simulink model "team_project_state_and_cds"  (R2023b)
settings: Solver=FixedStepAuto  StartTime=0.0  StopTime=inf  FixedStep=0.01  RelTol=1e-3  EnableMultiTasking=on
libraries: arduinolib x7
settings Model: ExtModeTrigDuration=2  Creator=권주성  LastModifiedBy=tkdle
settings OptimizationCC: EnhancedBackFolding=on  PassReuseOutputArgsAs=Individual arguments  ZeroExternalMemoryAtStartup=off  ZeroInternalMemoryAtStartup=off  MaxStackSize=64  OptimizeBlockOrder=speed  DifferentSizesBufferReuse=on  OptimizationCustomize=off  EfficientTunableParamExpr=on
settings DebuggingCC: ParameterTunabilityLossMsg=error
settings HardwareCC: ProdBitPerInt=16  ProdBitPerPointer=16  ProdBitPerSizeT=16  ProdBitPerPtrDiffT=16  ProdLargestAtomicFloat=None  ProdWordSize=8  ProdHWDeviceType=Atmel->AVR
settings SFSimCC: MATLABDynamicMemAlloc=off
settings RTWCC: Description=Embedded Coder  SystemTargetFile=ert.tlc  HardwareBoard=Arduino Mega ADK  TemplateMakefile=ert_default_tmf  Toolchain=Arduino AVR  BuildConfiguration=Faster Runs
settings CodeAppCC: ForceParamTrailComments=on  IgnoreCustomStorageClasses=off  OperatorAnnotations=on  SimulinkDataObjDesc=on  SFDataObjDesc=on  InsertBlockDesc=on
settings ERTTargetCC: SupportContinuousTime=on  SupportVariableSizeSignals=on  ExtModeTransport=3  ExtModeStaticAlloc=on  ExtModeAutomaticAllocSize=off  ExtModeStaticAllocSize=2048  ExtModeMexFile=ext_xcp  ExtModeIntrfLevel=Level2 - Open

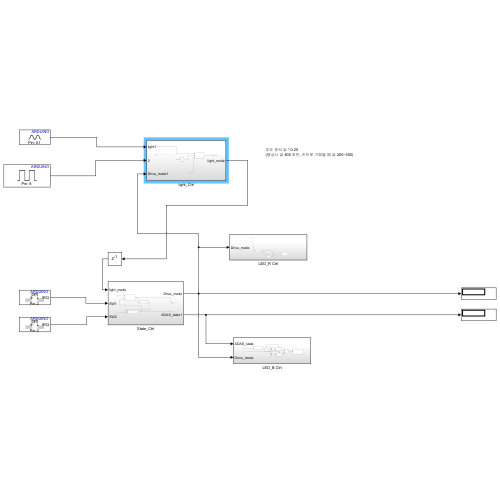
[thumbnail: Simulink's stored preview of the top-level diagram]
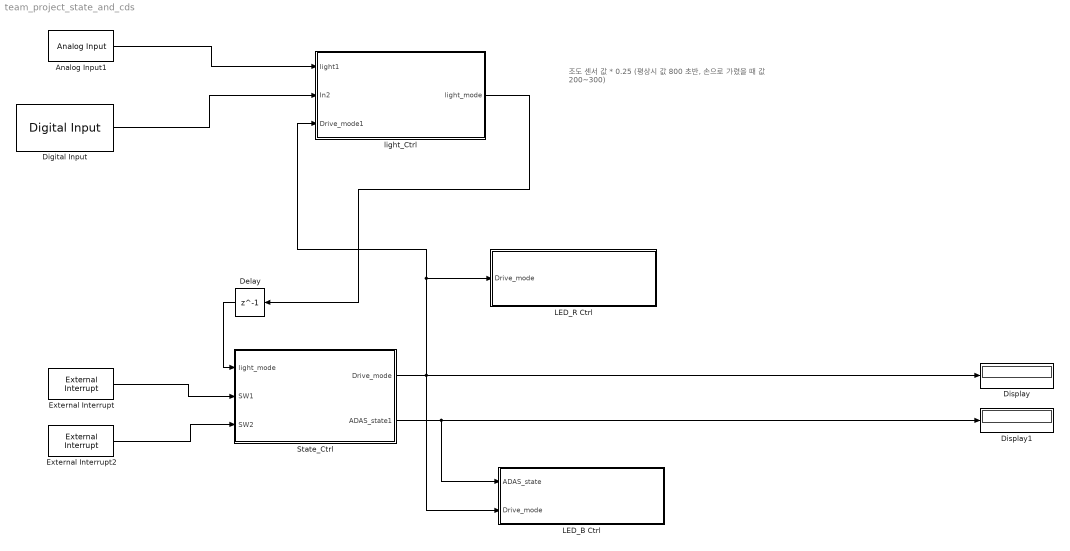
== system team_project_state_and_cds ==
  note: 조도 센서 값 * 0.25
      | (평상시 값 800 초반, 손으로 가렸을 때 값 200~300)
  Analog Input1 : arduinolib/Analog Input  pinNumber=1  ReadResultsOnly=off  ConversionTriggerSource=Software  ExternalTriggerType=uint32( 0 )  OutputDataType=uint16  EnableConversionCompleteNotify=off  EnableOuputStatus=off  SampleTime=-1  blockPlatform=arduino
  Delay : Delay  DelayLength=1
  Digital Input : arduinolib/Digital Input  pinNumber=8  mode=Default  Direction=input  SampleTime=0.1  blockPlatform=arduino
  Display : Display
  Display1 : Display
  External Interrupt : arduinolib/External Interrupt  Pin=2  PullUp=off  Mode=RISING  InterruptSimulationInput=off
  External Interrupt2 : arduinolib/External Interrupt  Pin=3  PullUp=off  Mode=RISING  InterruptSimulationInput=off
  LED_B Ctrl : Subsystem
  LED_R Ctrl : Subsystem
  State_Ctrl : Subsystem
  light_Ctrl : Subsystem
  wires:
  light_Ctrl/1(light_mode) -> Delay/1
  Digital Input/1 -> light_Ctrl/2(In2)
  Analog Input1/1 -> light_Ctrl/1(light1)
  Delay/1 -> State_Ctrl/1(light_mode)
  State_Ctrl/2(ADAS_state1) -> LED_B Ctrl/1(ADAS_state), Display1/1
  External Interrupt/1 -> State_Ctrl/2(SW1)
  External Interrupt2/1 -> State_Ctrl/3(SW2)
  State_Ctrl/1(Drive_mode) -> Display/1, light_Ctrl/3(Drive_mode1), LED_R Ctrl/1(Drive_mode), LED_B Ctrl/2(Drive_mode)

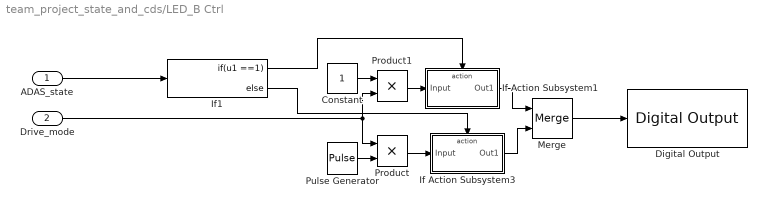
== system team_project_state_and_cds/LED_B Ctrl ==
  ADAS_state : Inport
  Drive_mode : Inport  Port=2
  Constant : Constant
  Digital Output : arduinolib/Digital Output  pinNumber=43  Direction=output  blockPlatform=arduino
  If Action Subsystem1 : Subsystem  TreatAsAtomicUnit=on
  If Action Subsystem3 : Subsystem  TreatAsAtomicUnit=on
  If1 : If  IfExpression=u1 ==1
  Merge : Merge
  Product : Product
  Product1 : Product
  Pulse Generator : DiscretePulseGenerator  PulseType=Time based  PulseWidth=50
  wires:
  If1/2 -> If Action Subsystem3/Action
  If Action Subsystem1/1(Out1) -> Merge/1
  ADAS_state/1 -> If1/1
  If1/1 -> If Action Subsystem1/Action
  Merge/1 -> Digital Output/1
  If Action Subsystem3/1(Out1) -> Merge/2
  Drive_mode/1 -> Product/1, Product1/2
  Pulse Generator/1 -> Product/2
  Constant/1 -> Product1/1
  Product1/1 -> If Action Subsystem1/1(Input)
  Product/1 -> If Action Subsystem3/1(Input)

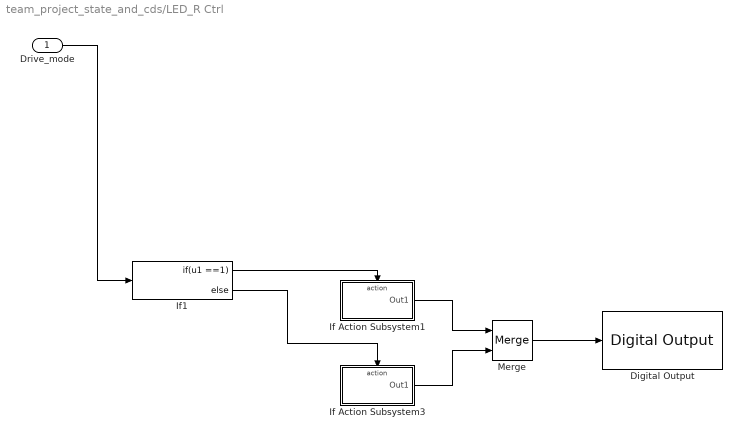
== system team_project_state_and_cds/LED_R Ctrl ==
  Drive_mode : Inport
  Digital Output : arduinolib/Digital Output  pinNumber=42  Direction=output  blockPlatform=arduino
  If Action Subsystem1 : Subsystem  TreatAsAtomicUnit=on
  If Action Subsystem3 : Subsystem  TreatAsAtomicUnit=on
  If1 : If  IfExpression=u1 ==1
  Merge : Merge
  wires:
  If1/2 -> If Action Subsystem3/Action
  If Action Subsystem1/1(Out1) -> Merge/1
  Drive_mode/1 -> If1/1
  If1/1 -> If Action Subsystem1/Action
  Merge/1 -> Digital Output/1
  If Action Subsystem3/1(Out1) -> Merge/2

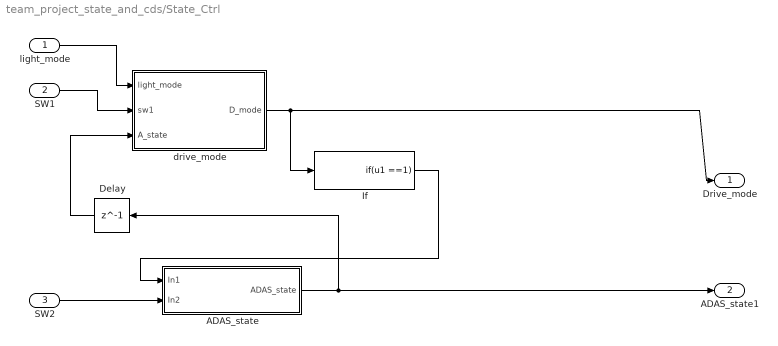
== system team_project_state_and_cds/State_Ctrl ==
  light_mode : Inport
  SW1 : Inport  Port=2
  SW2 : Inport  Port=3
  ADAS_state : Subsystem
  Delay : Delay  DelayLength=1
  If : If  IfExpression=u1 ==1  ShowElse=off
  drive_mode : Subsystem
  Drive_mode : Outport
  ADAS_state1 : Outport  Port=2
  wires:
  If/1 -> ADAS_state/1(In1)
  drive_mode/1(D_mode) -> If/1, Drive_mode/1
  SW2/1 -> ADAS_state/2(In2)
  ADAS_state/1(ADAS_state) -> Delay/1, ADAS_state1/1
  SW1/1 -> drive_mode/2(sw1)
  Delay/1 -> drive_mode/3(A_state)
  light_mode/1 -> drive_mode/1(light_mode)

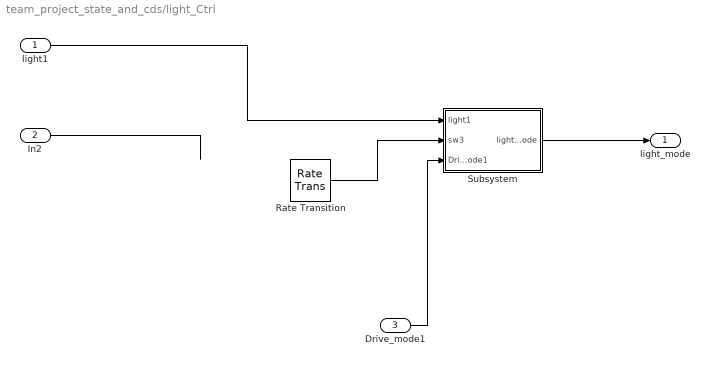
== system team_project_state_and_cds/light_Ctrl ==
  light1 : Inport
  In2 : Inport  Port=2
  Drive_mode1 : Inport  Port=3
  Rate Transition : RateTransition  Integrity=off  OutPortSampleTime=0.5
  Subsystem : Subsystem
  light_mode : Outport
  wires:
  ? -> Rate Transition/1
  In2/1 -> ?
  Rate Transition/1 -> Subsystem/2(sw3)
  Drive_mode1/1 -> Subsystem/3(Drive_mode1)
  light1/1 -> Subsystem/1(light1)
  Subsystem/1(light_mode) -> light_mode/1

== system team_project_state_and_cds/LED_B Ctrl/If Action Subsystem1 ==
  Input : Inport
  Action Port : ActionPort
  Out1 : Outport
  wires:
  Input/1 -> Out1/1

== system team_project_state_and_cds/LED_B Ctrl/If Action Subsystem3 ==
  Input : Inport
  Action Port : ActionPort
  Out1 : Outport
  wires:
  Input/1 -> Out1/1

== system team_project_state_and_cds/LED_R Ctrl/If Action Subsystem1 ==
  Action Port : ActionPort
  Constant : Constant
  Out1 : Outport
  wires:
  Constant/1 -> Out1/1

== system team_project_state_and_cds/LED_R Ctrl/If Action Subsystem3 ==
  Action Port : ActionPort
  Constant : Constant  Value=0
  Out1 : Outport
  wires:
  Constant/1 -> Out1/1

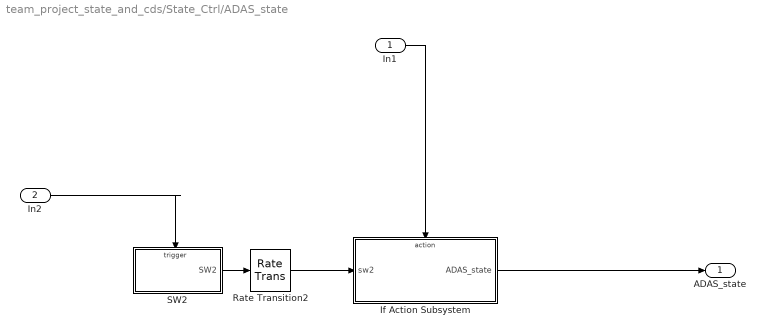
== system team_project_state_and_cds/State_Ctrl/ADAS_state ==
  In1 : Inport
  In2 : Inport  Port=2
  If Action Subsystem : Subsystem  TreatAsAtomicUnit=on
  Rate Transition2 : RateTransition  Integrity=off
  SW2 : Subsystem
  ADAS_state : Outport
  wires:
  Rate Transition2/1 -> If Action Subsystem/1(sw2)
  SW2/1(SW2) -> Rate Transition2/1
  In1/1 -> If Action Subsystem/Action
  In2/1 -> SW2/Trigger
  If Action Subsystem/1(ADAS_state) -> ADAS_state/1

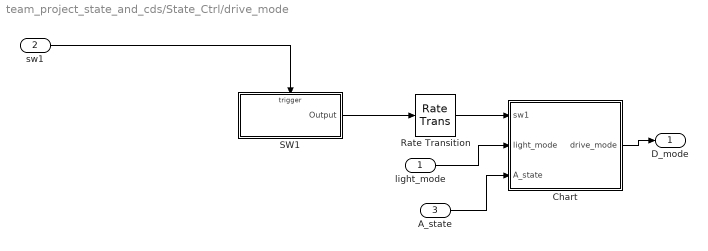
== system team_project_state_and_cds/State_Ctrl/drive_mode ==
  light_mode : Inport
  sw1 : Inport  Port=2
  A_state : Inport  Port=3
  Chart : Stateflow chart  TreatAsAtomicUnit=on
  Rate Transition : RateTransition  Integrity=off
  SW1 : Subsystem
  D_mode : Outport
  wires:
  SW1/1(Output) -> Rate Transition/1
  Rate Transition/1 -> Chart/1(sw1)
  Chart/1(drive_mode) -> D_mode/1
  sw1/1 -> SW1/Trigger
  A_state/1 -> Chart/3(A_state)
  light_mode/1 -> Chart/2(light_mode)

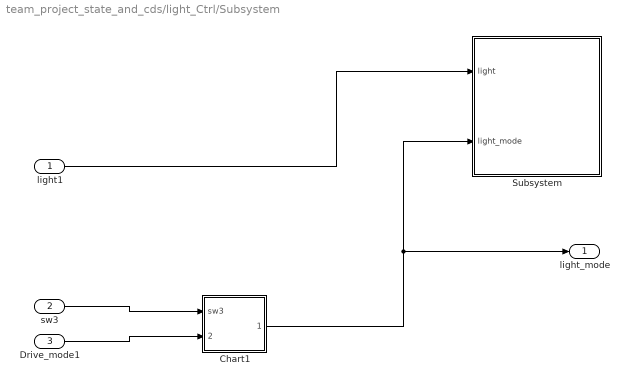
== system team_project_state_and_cds/light_Ctrl/Subsystem ==
  light1 : Inport
  sw3 : Inport  Port=2
  Drive_mode1 : Inport  Port=3
  Chart1 : Stateflow chart  TreatAsAtomicUnit=on
  Subsystem : Subsystem
  light_mode : Outport
  wires:
  Chart1/1(light_mode) -> Subsystem/2(light_mode), light_mode/1
  light1/1 -> Subsystem/1(light)
  sw3/1 -> Chart1/1(sw3)
  Drive_mode1/1 -> Chart1/2(Drive_mode)

== system team_project_state_and_cds/State_Ctrl/ADAS_state/If Action Subsystem ==
  sw2 : Inport
  Action Port : ActionPort
  Chart : Stateflow chart  TreatAsAtomicUnit=on
  ADAS_state : Outport
  wires:
  sw2/1 -> Chart/1(sw2)
  Chart/1(ADAS_state) -> ADAS_state/1

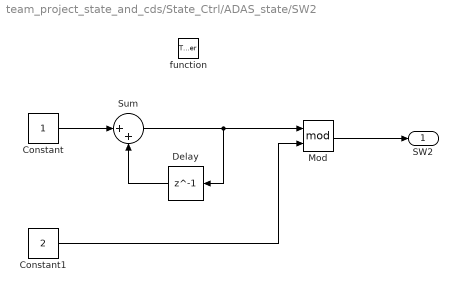
== system team_project_state_and_cds/State_Ctrl/ADAS_state/SW2 ==
  function : TriggerPort  TriggerType=function-call  VariantControl=(inherit)
  Constant : Constant
  Constant1 : Constant  Value=2
  Delay : Delay  DelayLength=1  InitialCondition=0
  Mod : Math  Operator=mod
  Sum : Sum  Inputs=|++
  SW2 : Outport
  wires:
  Sum/1 -> Delay/1, Mod/1
  Constant1/1 -> Mod/2
  Mod/1 -> SW2/1
  Constant/1 -> Sum/1
  Delay/1 -> Sum/2

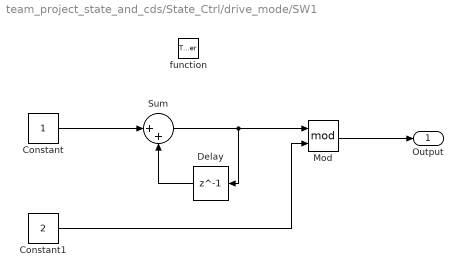
== system team_project_state_and_cds/State_Ctrl/drive_mode/SW1 ==
  function : TriggerPort  TriggerType=function-call  VariantControl=(inherit)
  Constant : Constant
  Constant1 : Constant  Value=2
  Delay : Delay  DelayLength=1
  Mod : Math  Operator=mod
  Sum : Sum  Inputs=|++
  Output : Outport
  wires:
  Constant/1 -> Sum/1
  Sum/1 -> Delay/1, Mod/1
  Constant1/1 -> Mod/2
  Delay/1 -> Sum/2
  Mod/1 -> Output/1

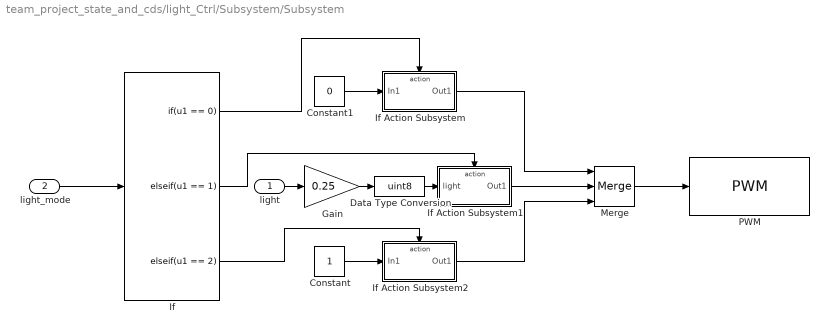
== system team_project_state_and_cds/light_Ctrl/Subsystem/Subsystem ==
  light : Inport
  light_mode : Inport  Port=2
  Constant : Constant
  Constant1 : Constant  Value=0
  Data Type Conversion : DataTypeConversion  OutDataTypeStr=uint8  SaturateOnIntegerOverflow=off  RndMeth=Floor
  Gain : Gain  Gain=0.25
  If : If  IfExpression=u1 == 0  ElseIfExpressions=u1 == 1, u1 == 2  ShowElse=off
  If Action Subsystem : Subsystem  TreatAsAtomicUnit=on
  If Action Subsystem1 : Subsystem  TreatAsAtomicUnit=on
  If Action Subsystem2 : Subsystem  TreatAsAtomicUnit=on
  Merge : Merge  Inputs=3
  PWM : arduinolib/PWM  pinNumber=9  frequencyType=Default  desiredFrequency=490.2  achievableFrequency=490.2
  wires:
  light_mode/1 -> If/1
  If/1 -> If Action Subsystem/Action
  If/2 -> If Action Subsystem1/Action
  If/3 -> If Action Subsystem2/Action
  Constant1/1 -> If Action Subsystem/1(In1)
  Constant/1 -> If Action Subsystem2/1(In1)
  If Action Subsystem/1(Out1) -> Merge/1
  If Action Subsystem1/1(Out1) -> Merge/2
  If Action Subsystem2/1(Out1) -> Merge/3
  Merge/1 -> PWM/1
  light/1 -> Gain/1
  Gain/1 -> Data Type Conversion/1
  Data Type Conversion/1 -> If Action Subsystem1/1(light)

== system team_project_state_and_cds/light_Ctrl/Subsystem/Subsystem/If Action Subsystem ==
  In1 : Inport
  Action Port : ActionPort
  Out1 : Outport
  wires:
  In1/1 -> Out1/1

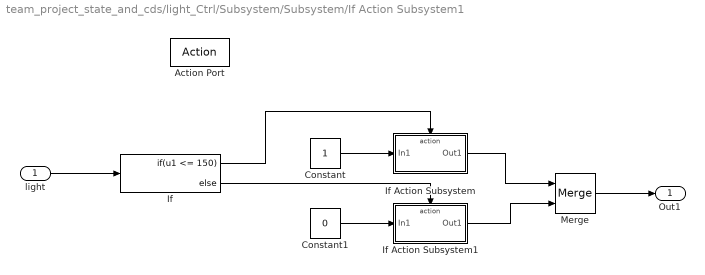
== system team_project_state_and_cds/light_Ctrl/Subsystem/Subsystem/If Action Subsystem1 ==
  light : Inport
  Action Port : ActionPort
  Constant : Constant
  Constant1 : Constant  Value=0
  If : If  IfExpression=u1 <= 150
  If Action Subsystem : Subsystem  TreatAsAtomicUnit=on
  If Action Subsystem1 : Subsystem  TreatAsAtomicUnit=on
  Merge : Merge
  Out1 : Outport
  wires:
  light/1 -> If/1
  Constant/1 -> If Action Subsystem/1(In1)
  Constant1/1 -> If Action Subsystem1/1(In1)
  If/1 -> If Action Subsystem/Action
  If/2 -> If Action Subsystem1/Action
  If Action Subsystem/1(Out1) -> Merge/1
  If Action Subsystem1/1(Out1) -> Merge/2
  Merge/1 -> Out1/1

== system team_project_state_and_cds/light_Ctrl/Subsystem/Subsystem/If Action Subsystem2 ==
  In1 : Inport
  Action Port : ActionPort
  Out1 : Outport
  wires:
  In1/1 -> Out1/1

== system team_project_state_and_cds/light_Ctrl/Subsystem/Subsystem/If Action Subsystem1/If Action Subsystem ==
  In1 : Inport
  Action Port : ActionPort
  Out1 : Outport
  wires:
  In1/1 -> Out1/1

== system team_project_state_and_cds/light_Ctrl/Subsystem/Subsystem/If Action Subsystem1/If Action Subsystem1 ==
  In1 : Inport
  Action Port : ActionPort
  Out1 : Outport
  wires:
  In1/1 -> Out1/1

== stateflow chart team_project_state_and_cds/State_Ctrl/ADAS_state/If Action Subsystem/Chart ==
  state adas_off
    en,du:
    ADAS_state = sw2;
    state_2 = sw2;
  state adas_on
    en,du:
    ADAS_state = sw2;
    state_2 =sw2;
  (default) -> adas_off
  adas_off -> adas_on : [state_2 ~= sw2]
  adas_on -> adas_off : [state_2 ~= sw2]
  data: sw2 input; state_2 local; ADAS_state output

== stateflow chart team_project_state_and_cds/State_Ctrl/drive_mode/Chart ==
  state Drive_off
    en, du:
    drive_mode = 0;
    state_1 = sw1;
  state Drive_on
    en,du:
    drive_mode =1;
    state_1 = sw1;
    ADAS_state = A_state;
    Light_state = light_mode;
  (default) -> Drive_off
  Drive_off -> Drive_on : [state_1 ~= sw1]
  Drive_on -> Drive_off : [(state_1~=sw1) && (ADAS_state == 0) && (Light_state == 0)]
  data: sw1 input; light_mode input; state_1 local; drive_mode output; A_state input; ADAS_state local; Light_state local

== stateflow chart team_project_state_and_cds/light_Ctrl/Subsystem/Chart1 ==
  state light_auto
    en, du:
    light_mode = 1;
    state_1 = sw3;
  state light_off
    en, du:
    light_mode =0;
    state_1 = sw3;
  state light_on
    en,du:
    light_mode =2;
    state_1 = sw3;
  light_auto -> (junction 15) : [(state_1 ~= sw3) && (Drive_mode == 1)]
  (junction 12) -> light_auto
  (junction 15) -> light_on
  light_off -> (junction 12) : [(state_1 ~= sw3) && (Drive_mode == 1)]
  (default) -> light_off
  light_on -> light_off : [(state_1 ~= sw3) && (Drive_mode == 1)]
  data: sw3 input; Drive_mode input; state_1 local; light_mode output
